simulink model "Vehicle_Model_WIP"  (R2019b)
settings: Solver=FixedStepDiscrete  StartTime=0.0  StopTime=Simulink.t_end  FixedStep=Simulink.dt  RelTol=1e-3
undefined symbols (not defined in the file): BRK, BTRRAD, CHLR, CHRG, DCDC, DiscIntNeverNeededParam, FAN, INV, MTR, PTRAD, PUMP, Settings, TRSM, Vehicle, VHCL, WHL
libraries: simulink x8, EV_cooling x6, EV_VLD x5, EV_ePWT x5
(part 1 of 5)
settings Model: SimulationMode=accelerator  Creator=matteo.yon  LastModifiedBy=matteo.paganini
settings DataIOCC: ReturnWorkspaceOutputs=off
settings DebuggingCC: ArithmeticOperatorsInVariantConditions=warning
settings SFSimCC: SimUseLocalCustomCode=off  CustomCodeUndefinedFunction=UseInterfaceOnly
settings RTWCC: RTWUseLocalCustomCode=off

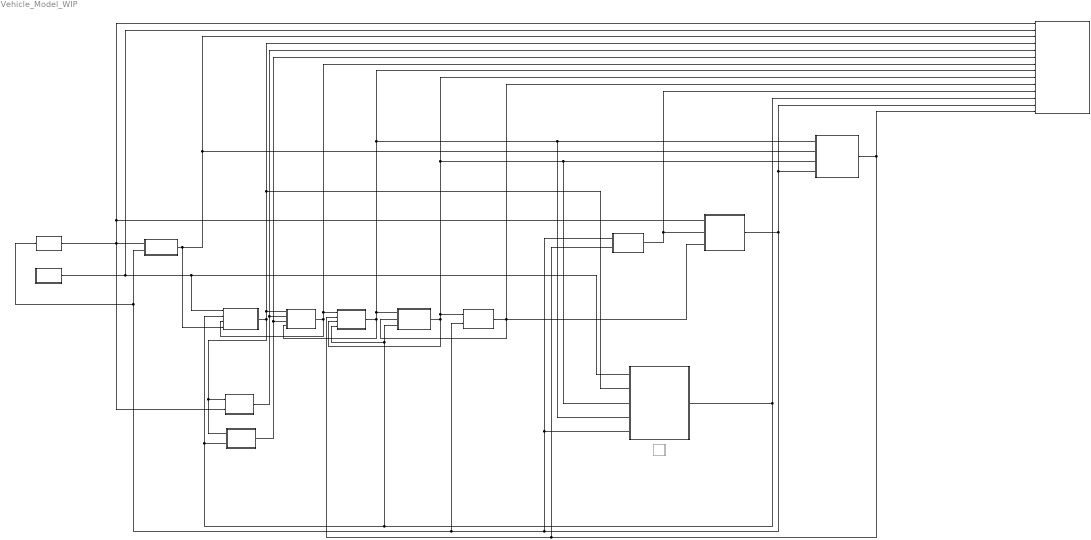
== system Vehicle_Model_WIP ==
  note: Cooling system
  note: Plot Results and Data Logging
  note: Electric Motor
  note: Inverter
  note: Initialization
  note: Battery Pack
  note: Model Input (speed cycle)
  note: Vehicle Longitudinal Dynamics
  note: Driver
  note: Transmission
  note: Electric Power Train Model
  note: Brake system
  note: Vehicle Control Unit
  note: DC Line
  note: DCDC
  note: Electric Vehicle Model
  note: Charger
  BRK : Subsystem
  BTR : Subsystem
  CHRG : Subsystem
  CS : Subsystem
  DC : Subsystem
  DCDC : Subsystem
  DRV : Subsystem
  INIT : Subsystem
  INPT : Subsystem
  INV : Subsystem
  MTR : Subsystem
  Plot Results and Data Logging : Subsystem
  TRSM : Subsystem
  VCU : Subsystem
  VLD : Subsystem
  old cooling : Subsystem  Commented=on
  wires:
  INPT/1(INPT) -> Plot Results and Data Logging/1(INPT), VLD/1(INPT), CHRG/2(INPT), DRV/1(INPT)  "INPT"
  BTR/1(BTR) -> DCDC/1(BTR), CHRG/1(BTR), DC/1(BTR), Plot Results and Data Logging/4(BTR), CS/2(BTR)
  DRV/1(DRV) -> BTR/4(DRV), Plot Results and Data Logging/3(DRV), VCU/2(DRV)  "DRV"
  INV/1(INV) -> MTR/1(INV), Plot Results and Data Logging/8(INV), CS/4(INV), VCU/1(INV), DC/4(INV)
  MTR/1(MTR) -> Plot Results and Data Logging/9(MTR), CS/3(MTR), VCU/3(MTR), TRSM/1(MRT), INV/3(MTR)
  TRSM/1(TRSM) -> Plot Results and Data Logging/10(TRSM), VLD/3(TRSM), MTR/2(TRSM)  "TRSM"
  BRK/1(BRK) -> Plot Results and Data Logging/11(BRK), VLD/2(BRK)
  INIT/1(INIT) -> CS/1(INIT), BTR/1(INIT), Plot Results and Data Logging/2(INIT)  "INIT"
  DC/1(DC) -> BTR/3(DC), Plot Results and Data Logging/7(DC), INV/1(DC)
  VLD/1(VLD) -> Plot Results and Data Logging/13(VLD), VCU/4(VLD), TRSM/2(VLD), DRV/2(VLD), INPT/1(VLD), BRK/1(VLD), CS/5(VLD)  "LVD"
  VCU/1(VCU) -> BRK/2(VCU), INV/2(VCU), Plot Results and Data Logging/14(VCU)  "VCU"
  DCDC/1(DCDC) -> Plot Results and Data Logging/6(DCDC), DC/3(DCDC)
  CHRG/1(CHRG) -> DC/2(CHRG), Plot Results and Data Logging/5(CHRG)
  CS/1(CS) -> Plot Results and Data Logging/12(CS), INV/4(CS), MTR/3(CS), BTR/2(CS), DCDC/2(CS)

== system Vehicle_Model_WIP/BRK ==
  note: Rear Brake
  note: Front Brake
  note: Inverter model:
      | Input: Brake cmd from VCU model.
      | Output: Brake torque.
  VLD : Inport
  VCU : Inport  Port=2
  Add3 : Sum
  Bus Creator : BusCreator  Inputs=6
  Bus Selector2 : BusSelector  OutputSignals=VLD_nWhlFr_rpm,VLD_nWhlRr_rpm,VLD_vActVhcl_kph
  Bus Selector3 : BusSelector  OutputSignals=VCU_rBrkCmdFrt,VCU_rBrkCmdRr
  Constant1 : Constant  Value=Simulink.INIT_TSys_degC
  Constant2 : Constant  Value=Simulink.INIT_TSys_degC
  Discrete-Time Integrator : DiscreteIntegrator  IntegratorMethod=Integration: Trapezoidal  gainval=1e-3/3600  SampleTime=-1  ICPrevOutput=DiscIntNeverNeededParam  ICPrevScaledInput=DiscIntNeverNeededParam
  Front BRAKE : EV_VLD/BRAKE  MxTrq_Nm=BRK.Front.Mx_Torque_Nm/2  eff=BRK.Front.Eff_BrkSys  HC_disc=BRK.Front.Cdisc_JpK  T_env_degC=Simulink.INIT_TEnv_degC  R_StoC_KpW=0.0035*0.8  HTC_v_bp=BRK.Front.HTC_v_bp  HTC_map=BRK.Front.HTC_map
      settings: SourceProductName=EV_lib
  Gain{1..4} (4 alike) : Gain  Gain=2
  Rear BRAKE : EV_VLD/BRAKE  MxTrq_Nm=BRK.Rear.Mx_Torque_Nm/2  eff=BRK.Rear.Eff_BrkSys  HC_disc=BRK.Rear.Cdisc_JpK  T_env_degC=Simulink.INIT_TEnv_degC  R_StoC_KpW=0.0035*0.8  HTC_v_bp=BRK.Rear.HTC_v_bp  HTC_map=BRK.Rear.HTC_map
      settings: SourceProductName=EV_lib
  Scope1 : Scope  NumInputPorts=2
  BRK : Outport  VectorParamsAs1DForOutWhenUnconnected=off
  wires:
  Bus Creator/1 -> BRK/1
  VCU/1 -> Bus Selector3/1
  VLD/1 -> Bus Selector2/1
  [BRK_TActFrt_Nm] -> Bus Creator/1  "BRK_TActFrt_Nm"
  [BRK_TActRr_Nm] -> Bus Creator/2  "BRK_TActRr_Nm"
  Bus Selector2/1 -> [VLD_nWhlFr_rpm]  "<VLD_nWhlFr_rpm>"
  Bus Selector2/2 -> [VLD_nWhlRr_rpm]  "<VLD_nWhlRr_rpm>"
  Bus Selector3/2 -> [VCU_rBrkCmdRr]  "<VCU_rBrkCmdRr>"
  Bus Selector3/1 -> [VCU_rBrkCmdFrt]  "<VCU_rBrkCmdFrt>"
  [BRK_PwrFrt_W] -> Add3/1
  [BRK_PwrRr_W] -> Add3/2
  Add3/1 -> Discrete-Time Integrator/1, [BRK_Pwr_W]
  [BRK_Pwr_W] -> Bus Creator/3  "BRK_Pwr_W"
  Discrete-Time Integrator/1 -> [BRK_E_kWh]
  [BRK_E_kWh] -> Bus Creator/4  "BRK_E_kWh"
  Front BRAKE/2 -> Gain2/1
  Front BRAKE/1 -> Gain3/1
  [VLD_nWhlFr_rpm] -> Front BRAKE/2
  Bus Selector2/3 -> [VLD_vActVhcl_kph]  "<VLD_vActVhcl_kph>"
  [VLD_vActVhcl_kph] -> Front BRAKE/3
  Constant1/1 -> Front BRAKE/4
  Front BRAKE/3 -> Scope1/1, [BRK_TFrt_degC]
  Rear BRAKE/1 -> Gain1/1
  Rear BRAKE/3 -> [BRK_TRr_degC], Scope1/2
  Rear BRAKE/2 -> Gain4/1
  Constant2/1 -> Rear BRAKE/4
  [VLD_nWhlRr_rpm] -> Rear BRAKE/2
  [VLD_vActVhcl_kph] -> Rear BRAKE/3
  [BRK_TFrt_degC] -> Bus Creator/5  "BRK_TFrt_degC"
  [BRK_TRr_degC] -> Bus Creator/6  "BRK_TRr_degC"
  Gain2/1 -> [BRK_PwrFrt_W]
  Gain3/1 -> [BRK_TActFrt_Nm]
  [VCU_rBrkCmdFrt] -> Front BRAKE/1
  Gain1/1 -> [BRK_TActRr_Nm]
  Gain4/1 -> [BRK_PwrRr_W]
  [VCU_rBrkCmdRr] -> Rear BRAKE/1

== system Vehicle_Model_WIP/BTR ==
  INIT : Inport
  CS : Inport  Port=2
  DC : Inport  Port=3
  DRV : Inport  Port=4
  1-D Lookup Table1 : Lookup_n-D  NumberOfTableDimensions=1  BreakpointsForDimension1=[0 20 50 100]  Table=[0 0 1 1]  InternalRulePriority=Speed  RndMeth=Simplest  InputSameDT=on
  1-D Lookup Table2 : Lookup_n-D  NumberOfTableDimensions=1  BreakpointsForDimension1=[0 60 80 100]  Table=[250 250 0 0]*1e3  InternalRulePriority=Speed  RndMeth=Simplest  InputSameDT=on
  Battery : EV_ePWT/Battery  n_series=BTR.cell_p.n_series  n_parallel=BTR.cell_p.n_parallel  weight_ratio=0.7  C_cell_Ah=BTR.cell_p.capacity_nom  V_nominal=BTR.cell_p.voltage_nom  R_contact=0  V_low=BTR.cell_p.Vmin  V_up=BTR.cell_p.Vmax  R_th_KpW=BTR.cell_p.R_th  c_th=BTR.cell_p.c_th  weight=BTR.cell_p.weight  VoC_map=BTR.cell_p.VOC  VoC_SoC_bp=BTR.cell_p.SOC_bp_VOC  VoC_Temp_bp=BTR.cell_p.Temp_bp_VOC  VoC_C_bp=BTR.cell_p.C_bp  R0_map=BTR.cell_p.R0  R0_SoC_bp=BTR.cell_p.SOC_bp  R0_Temp_bp=BTR.cell_p.Temp_bp  R0_i_bp=BTR.cell_p.I_bp  R0_C_bp=BTR.cell_p.C_bp  R1_map=BTR.cell_p.R1  R1_SoC_bp=BTR.cell_p.SOC_bp  R1_Temp_bp=BTR.cell_p.Temp_bp  R1_i_bp=BTR.cell_p.I_bp  R1_C_bp=BTR.cell_p.C_bp  tau1_map=BTR.cell_p.tau  tau1_SoC_bp=BTR.cell_p.SOC_bp  tau1_Temp_bp=BTR.cell_p.Temp_bp  tau1_i_bp=BTR.cell_p.I_bp  tau1_C_bp=BTR.cell_p.C_bp  Limit_temp_bp=[-30 -10 0 55 57 58]  Limit_map=[0 0.2 1 1 0.2 0]  max_peak_crate=10  max_crate=5  peak_time=30
  Bus Creator : BusCreator  Inputs=13
  Bus Selector : BusSelector  OutputSignals=INIT_TSys_degC,INIT_SocBtr_Pct
  Bus Selector1 : BusSelector  OutputSignals=DC_PBtrReq_W
  Bus Selector2 : BusSelector  OutputSignals=CS_BTR_TWtrOut_degC,CS_BTR_dm_kgps
  Bus Selector3 : BusSelector  OutputSignals=DRV_FC_enable
  Delay1 : Delay  DelayLength=1
  Delay2 : Delay  DelayLength=1  InitialCondition=20000
  Divide : Product  Inputs=*/
  FuelCells : Subsystem
  Gain : Gain  Gain=100
  Gain1 : Gain  Gain=1/100
  Gain2 : Gain  Gain=1e-3
  Mux : Mux  Inputs=2
  Product : Product
  Scope : Scope  NumInputPorts=2
  Sum : Sum  Inputs=-+|
  Sum1 : Sum  Inputs=++|
  Tentativo picchi richiesta FC : Lookup_n-D  NumberOfTableDimensions=1  BreakpointsForDimension1=[0 40 45 100]  Table=[250 250 0 0]*1e3  InternalRulePriority=Speed  RndMeth=Simplest  InputSameDT=on
  Terminator : Terminator
  Terminator2 : Terminator
  To Workspace : ToWorkspace  VariableName=actPower_W  SaveFormat=Timeseries  SampleTime=-1
  reset_time : Constant  Value=1e6
  BTR : Outport  VectorParamsAs1DForOutWhenUnconnected=off
  wires:
  [INIT_SocBtr_Pct] -> Gain1/1
  [BTR_VPackEst_V] -> Bus Creator/2  "BTR_VPackEst_V"
  [BTR_iPackEst_A] -> Bus Creator/1  "BTR_iPackEst_A"
  [BTR_PPackEst_W] -> Bus Creator/3  "BTR_PPackEst_W"
  [BTR_SocPack_Ptc] -> Bus Creator/4  "BTR_SocPack_Ptc"
  [BTR_PMxDsch_W] -> Bus Creator/5  "BTR_PMxDsch_W"
  [BTR_PMxChrg_W] -> Bus Creator/6  "BTR_PMxChrg_W"
  [BTR_TMxCell_degC] -> Bus Creator/7  "BTR_TMxCell_degC"
  [BTR_TMxBsbr_C] -> Bus Creator/8  "BTR_TMxBsbr_C"
  [BTR_TWtrOut_degC] -> Bus Creator/9  "BTR_TWtrOut_degC"
  Bus Creator/1 -> BTR/1
  INIT/1 -> Bus Selector/1
  Bus Selector/2 -> [INIT_SocBtr_Pct]  "<INIT_SocBtr_Pct>"
  Bus Selector/1 -> [INIT_TSys_degC]  "<INIT_TSys_degC>"
  DC/1 -> Bus Selector1/1
  Bus Selector1/1 -> [DC_PBtrReq_W]  "<DC_PBtrReq_W>"
  CS/1 -> Bus Selector2/1
  Bus Selector2/1 -> [BCS_TWtrOut_degC]  "<CS_BTR_TWtrOut_degC>"
  Bus Selector2/2 -> [BCS_dm_kgps]  "<CS_BTR_dm_kgps>"
  Delay1/1 -> [BTR_PBtrReq_W], Battery/1
  Battery/3 -> [BTR_PPackEst_W]
  Battery/4 -> [BTR_iPackEst_A]
  Battery/6 -> Gain/1
  Battery/10 -> [BTR_PMxChrg_W]
  Battery/7 -> [BTR_TMxBsbr_C], [BTR_TMxCell_degC]
  Battery/5 -> [BTR_VPackEst_V]
  Gain/1 -> Scope/2, [BTR_SocPack_Ptc]  "HVB_SOC"
  [INIT_TSys_degC] -> Battery/3
  Battery/1 -> Terminator2/1
  Gain1/1 -> Battery/2
  Battery/2 -> [BTR_EPack_kWh]
  [BTR_EPack_kWh] -> Bus Creator/10  "BTR_EPack_kWh"
  reset_time/1 -> Battery/6
  Battery/11 -> [BTR_HR_pack_W]
  [BTR_HR_pack_W] -> Bus Creator/11  "BTR_HR_pack_W"
  [BCS_dm_kgps] -> Battery/4
  [BCS_TWtrOut_degC] -> Battery/5
  Battery/8 -> [BTR_TWtrOut_degC]
  [DC_PBtrReq_W] -> Sum/2
  Sum/1 -> Mux/2, Delay1/1  "HVB_P"
  FuelCells/1(actPower_W) -> To Workspace/1, Mux/1, [BTR_FCPower_W], Sum/1  "FC_P"
  [BTR_FCPower_W] -> Bus Creator/12  "BTR_FCPower_W"
  Battery/9 -> Product/2
  Sum1/1 -> [BTR_PMxDsch_W]
  [BTR_FCPower_W] -> Delay2/1
  Delay2/1 -> Sum1/1
  1-D Lookup Table2/1 -> FuelCells/1(reqPower_W)
  [BTR_SocPack_Ptc] -> 1-D Lookup Table2/1
  [BTR_PBtrReq_W] -> Bus Creator/13  "BTR_PBtrReq_W"
  Mux/1 -> Scope/1
  [BTR_SocPack_Ptc] -> 1-D Lookup Table1/1
  Product/1 -> Sum1/2
  1-D Lookup Table1/1 -> Product/1
  [BTR_EPack_kWh] -> Divide/2
  Divide/1 -> Terminator/1  "BTR_PDsch_C"
  [BTR_PPackEst_W] -> Gain2/1
  Gain2/1 -> Divide/1
  DRV/1 -> Bus Selector3/1
  Bus Selector3/1 -> [DRV_FC_enable]  "<DRV_FC_enable>"
  [DRV_FC_enable] -> FuelCells/2(DRV_FC_enable)

== system Vehicle_Model_WIP/CHRG ==
  note: Charger model (only efficiency).
      | Input: charge power.
      | Output: charge power to the DC line.
  BTR : Inport
  INPT : Inport  Port=2
  1-D Lookup Table : Lookup_n-D  NumberOfTableDimensions=1  BreakpointsForDimension1=[-20 0 5 90]  Table=-[250 350 450 450]  InternalRulePriority=Speed  RndMeth=Simplest  InputSameDT=on
  1/C : Gain  Gain=1/1516.15
  1/R_toair : Gain  Gain=1/0.5
  Abs : Abs
  Bus Creator : BusCreator  Inputs=3
  Bus Selector1 : BusSelector  OutputSignals=INPT_PwrChrg_W
  Bus Selector2 : BusSelector  OutputSignals=BTR_VPackEst_V,BTR_PMxChrg_W
  Constant3 : Constant  Value=CHRG.Efficiency
  Discrete-Time Integrator : DiscreteIntegrator  InitialConditionSource=external  InitialCondition=23  SampleTime=-1  ICPrevOutput=DiscIntNeverNeededParam  ICPrevScaledInput=DiscIntNeverNeededParam
  Divide1 : Product  Inputs=*/
  Divide2 : Product  Inputs=**
  Divide3 : Product  Inputs=*/
  Divide4 : Product  Inputs=*/
  MinMax1 : MinMax  Function=max  Inputs=3
  MinMax2 : MinMax  Function=max  Inputs=2
  R_joule : Gain  Gain=0.001
  Scope : Scope
  Scope1 : Scope
  Scope2 : Scope
  Square : Math  Operator=square  SignedPower=off  SaturateOnIntegerOverflow=on
  Subtract : Sum  Inputs=+-
  Subtract1 : Sum  Inputs=+-
  Subtract2 : Sum  Inputs=-+
  Switch : Switch  Criteria=u2 > Threshold  Threshold=1e4
  T_ambient : Constant  Value=Simulink.INIT_TEnv_degC
  T_ref : Constant  Value=90
  CHRG : Outport  VectorParamsAs1DForOutWhenUnconnected=off
  wires:
  [CHRG_Pwr_W] -> Bus Creator/1  "CHRG_Pwr_W"
  Bus Selector1/1 -> [INPT_PwrChrg_W]  "<INPT_PwrChrg_W>"
  Bus Creator/1 -> CHRG/1
  INPT/1 -> Bus Selector1/1
  Constant3/1 -> [CHRG_rEff]
  [T_port_degC] -> Bus Creator/3  "CHRG_Tport_degC"
  BTR/1 -> Bus Selector2/1
  Bus Selector2/1 -> [BTR_VPackEst_V]  "<BTR_VPackEst_V>"
  Square/1 -> R_joule/1
  [T_port_degC] -> Subtract1/1
  1/R_toair/1 -> Subtract/2
  T_ambient/1 -> Discrete-Time Integrator/2, Subtract1/2
  Subtract1/1 -> 1/R_toair/1  "q_dot"
  R_joule/1 -> Subtract/1
  Subtract/1 -> 1/C/1  "q_dot"
  1/C/1 -> Discrete-Time Integrator/1  "dT"
  Discrete-Time Integrator/1 -> Scope2/1, [T_port_degC]  "T"
  Bus Selector2/2 -> [BTR_PMxChrg_W]  "<BTR_PMxChrg_W>"
  [CHRG_iAct_A] -> Square/1  "iChrg_A"
  [CHRG_iAct_A] -> Bus Creator/2  "CHRG_iAct_A"
  [T_port_degC] -> Subtract2/1
  T_ref/1 -> Subtract2/2
  Subtract2/1 -> 1-D Lookup Table/1
  [BTR_VPackEst_V] -> Divide1/2
  [BTR_PMxChrg_W] -> Divide1/1
  Divide1/1 -> MinMax1/1  "iMxChrg_A"
  1-D Lookup Table/1 -> MinMax1/2
  MinMax1/1 -> [CHRG_iAct_A], Scope1/1
  Divide2/1 -> [CHRG_Pwr1_W]
  [CHRG_iAct_A] -> Divide2/1
  [BTR_VPackEst_V] -> Divide2/2
  [INPT_PwrChrg_W] -> Divide3/1
  [BTR_VPackEst_V] -> Divide3/2
  Divide3/1 -> MinMax1/3  "INPT_iChrg_A"
  [CHRG_Pwr1_W] -> Switch/1, Abs/1
  Abs/1 -> Switch/2
  Switch/1 -> Scope/1, [CHRG_Pwr_W]
  [INPT_PwrChrg_W] -> Divide4/1
  [CHRG_rEff] -> Divide4/2
  Divide4/1 -> MinMax2/1
  MinMax2/1 -> Switch/3
  [BTR_PMxChrg_W] -> MinMax2/2

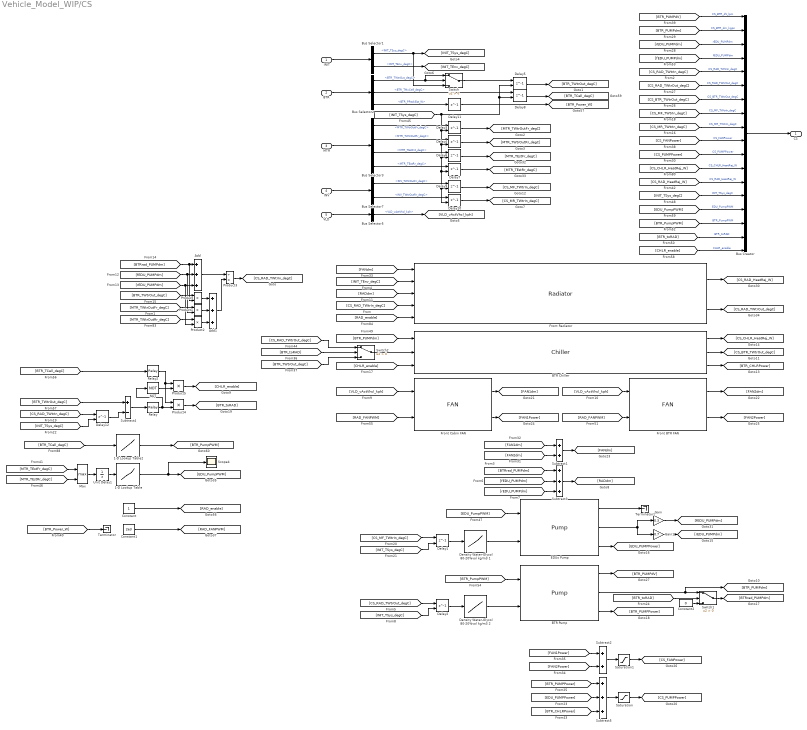
== system Vehicle_Model_WIP/CS ==
  INIT : Inport
  BTR : Inport  Port=2
  MTR : Inport  Port=3
  INV : Inport  Port=4
  VLD : Inport  Port=5
  1-D Lookup Table : Lookup_n-D  NumberOfTableDimensions=1  BreakpointsForDimension1=[0 60 100 120 150]  Table=[1000 1000 3500 5500 5500]  InternalRulePriority=Speed  RndMeth=Simplest  InputSameDT=on
  1-D Lookup Table2 : Lookup_n-D  NumberOfTableDimensions=1  BreakpointsForDimension1=[0 35 50 55 70]  Table=[2000 2000 4000 5500 5500]  InternalRulePriority=Speed  RndMeth=Simplest  InputSameDT=on
  Add : Sum  Inputs=+++
  Add1 : Sum  Inputs=+++
  BTR Chiller : EV_cooling/Chiller  dm_water_bp=(0:0.05:0.25)'  T_water_bp=0:10:40  HR_map=[0,0,0,0,0;0,300,600,900,0;0,600,1200,1800,0;0,900,1800,2700,0;0,1200,2400,3600,0;0,1500,3000,4500,0]  COP=2.5
      settings: SourceProductName=EV_lib
  BTR Pump : EV_cooling/Pump  RPM_bp=PUMP.Front.BCS_RPM_bp1  dV_map=PUMP.Front.BCS_dV  power_map=PUMP.Front.BCS_power
      settings: SourceProductName=EV_lib
  Bus Creator : BusCreator  Inputs=18
  Bus Selector1 : BusSelector  OutputSignals=INIT_TSys_degC,INIT_TEnv_degC
  Bus Selector2 : BusSelector  OutputSignals=BTR_TWtrOut_degC,BTR_TMxCell_degC,BTR_PPackEst_W
  Bus Selector3 : BusSelector  OutputSignals=MTR_TWtrOutFr_degC,MTR_TWtrOutRr_degC,MTR_TEstFrt_degC,MTR_TEstRr_degC
  Bus Selector5 : BusSelector  OutputSignals=VLD_vActVhcl_kph
  Bus Selector7 : BusSelector  OutputSignals=INV_TWtrOutFr_degC,INV_TWtrOutRr_degC
  Constant : Constant
  Constant1 : Constant  Value=2e3
  Constant2 : Constant  Value=0
  Delay{1..10,12} (11 alike) : Delay  DelayLength=1  InitialConditionSource=Input port
      settings: InputPortMap=u0,p4
  Delay11 : Delay  DelayLength=1
  Density Water-Glycol 80-20%vol kg/m3 1 : Lookup_n-D  NumberOfTableDimensions=1  BreakpointsForDimension1=[-45.56 -17.78 10 37.77 65.55 93.33 121.11 148.88 176.66]  Table=[1.02e+03 1.03e+03 1.03e+03 1.02e+03 9.99e+02 9.85e+02 9.63e+02 9.38e+02 9.11e+02]  ExtrapMethod=Clip  RndMeth=Simplest  InputSameDT=on
  Density Water-Glycol 80-20%vol kg/m3 2 : Lookup_n-D  NumberOfTableDimensions=1  BreakpointsForDimension1=[-45.56 -17.78 10 37.77 65.55 93.33 121.11 148.88 176.66]  Table=[1.02e+03 1.03e+03 1.03e+03 1.02e+03 9.99e+02 9.85e+02 9.63e+02 9.38e+02 9.11e+02]  ExtrapMethod=Clip  RndMeth=Simplest  InputSameDT=on
  EDUs Pump : EV_cooling/Pump  RPM_bp=PUMP.Front.PWT_RPM_bp1  dV_map=PUMP.Front.PWT_dV  power_map=PUMP.Front.PWT_power
      settings: SourceProductName=EV_lib
  Front BTR FAN : EV_cooling/FAN  speed_bp=FAN.Front.f15_V_bp  RPM_bp=FAN.Front.f15_RPM_bp  dm_map=FAN.Front.f15_dm_air  power_map=FAN.Front.f15_power
      settings: SourceProductName=EV_lib
  Front Cabin FAN : EV_cooling/FAN  speed_bp=FAN.Front.f11_V_bp  RPM_bp=FAN.Front.f11_RPM_bp  dm_map=FAN.Front.f11_dm_air  power_map=FAN.Front.f11_power
      settings: SourceProductName=EV_lib
  Front Radiator : EV_cooling/Radiator  dm_water_bp=RAD.Front.FC_dmw_bp  dm_air_bp=RAD.Front.FC_dma_bp  normHR_map=RAD.Front.FC_normHR  FrontSurf=RAD.Front.ABTR_m2
      settings: SourceProductName=EV_lib
  Gain : Gain  Gain=0.3
  Gain1 : Gain  Gain=0.7
  Max : MinMax  Function=max  Inputs=2
  NOT : Logic  Operator=NOT  IconShape=distinctive  AllPortsSameDT=off  OutDataTypeStr=boolean
  Product{,1..2,4..5} (5 alike) : Product
  Product3 : Product  Inputs=/*
  Relay : Relay  OnSwitchValue=2  OffSwitchValue=-2
  Relay2 : Relay  OnSwitchValue=31  OffSwitchValue=29
  Saturation : Saturate  UpperLimit=0  LowerLimit=0
  Saturation1 : Saturate  UpperLimit=0  LowerLimit=0
  Scope4 : Scope
  Subtract1 : Sum
  Subtract2 : Sum
  Subtract3 : Sum  Inputs=+++
  Subtract4 : Sum  Inputs=+-
  Subtract5 : Sum  Inputs=+++
  Switch : Switch  Criteria=u2 > Threshold
  Switch1 : Switch  Criteria=u2 > Threshold
  Switch2 : Switch  Criteria=u2 > Threshold
  Terminator : Terminator
  Terminator2 : Terminator
  Unit Delay1 : UnitDelay  InitialCondition=Settings.INIT_TSys_degC  SampleTime=-1  HasFrameUpgradeWarning=on
  CS : Outport
  wires:
  Bus Selector1/2 -> [INIT_TEnv_degC]  "<INIT_TEnv_degC>"
  INIT/1 -> Bus Selector1/1
  Bus Selector1/1 -> Switch/3, [INIT_TSys_degC]  "<INIT_TSys_degC>"
  BTR/1 -> Bus Selector2/1
  MTR/1 -> Bus Selector3/1
  Bus Selector5/1 -> [VLD_vActVhcl_kph]  "<VLD_vActVhcl_kph>"
  VLD/1 -> Bus Selector5/1
  [CS_RAD_TWtrIn_degC] -> Front Radiator/4
  Bus Creator/1 -> CS/1
  [CS_MR_TWtrIn_degC] -> Bus Creator/9  "CS_MR_TWtrIn_degC"
  [CS_MF_TWtrIn_degC] -> Bus Creator/8  "CS_MF_TWtrIn_degC"
  [INIT_TSys_degC] -> Delay1/2
  [CS_MF_TWtrIn_degC] -> Delay1/1
  Delay1/1 -> Density Water-Glycol 80-20%vol kg/m3 1/1
  [EDU_PumpPWM] -> EDUs Pump/1
  EDUs Pump/2 -> Gain/1, Gain1/1
  EDUs Pump/3 -> [EDU_PUMPPower]
  BTR Pump/3 -> [BTR_PUMPPower]
  Delay2/1 -> Density Water-Glycol 80-20%vol kg/m3 2/1
  [INIT_TSys_degC] -> Delay2/2
  [CS_RAD_TWtrOut_degC] -> Delay2/1
  [CS_RAD_TWtrOut_degC] -> Bus Creator/6  "CS_RAD_TWtrOut_degC"
  [rEDU_PUMPdm] -> Bus Creator/3  "rEDU_PUMPdm"
  [BTR_PUMPdm] -> Bus Creator/2  "CS_BTR_dm_kgps"
  [BTR_PUMPPower] -> Subtract5/1
  [EDU_PUMPPower] -> Subtract5/2
  Subtract5/1 -> Saturation/1
  [CS_PUMPPower] -> Bus Creator/11  "CS_PUMPPower"
  Front BTR FAN/1 -> [FAN2dm]
  [FAN1dm] -> Subtract1/1
  [FAN2dm] -> Subtract1/2
  Subtract1/1 -> [FANdm]
  [FANdm] -> Front Radiator/1
  Front Radiator/1 -> [CS_RAD_HeatRej_W]
  Front BTR FAN/2 -> [FAN2Power]
  [FAN1Power] -> Subtract2/1
  [FAN2Power] -> Subtract2/2
  Subtract2/1 -> Saturation1/1
  [CS_FANPower] -> Bus Creator/10  "CS_FANPower"
  [BTR_PUMPdV] -> Bus Creator/1  "CS_BTR_dV_lpm"
  Bus Selector3/1 -> Delay3/1  "<MTR_TWtrOutFr_degC>"
  Bus Selector3/2 -> Delay4/1  "<MTR_TWtrOutRr_degC>"
  Delay3/1 -> [MTR_TWtrOutFr_degC]
  Delay4/1 -> [MTR_TWtrOutRr_degC]
  [CS_RAD_HeatRej_W] -> Bus Creator/13  "CS_RAD_HeatRej_W"
  Front Cabin FAN/2 -> [FAN1Power]
  Front Cabin FAN/1 -> [FAN1dm]
  EDUs Pump/1 -> Terminator2/1
  BTR Pump/1 -> [BTR_PUMPdV]
  Switch/1 -> Delay5/1
  [INIT_TSys_degC] -> Delay8/2, Delay5/2, Delay10/2, Delay9/2, Delay7/2, Delay6/2, Delay4/2, Delay3/2
  Delay5/1 -> [BTR_TWtrOut_degC]
  Delay7/1 -> [MTR_TEstRr_degC]
  Delay6/1 -> [MTR_TEstFr_degC]
  Bus Selector3/4 -> Delay7/1  "<MTR_TEstRr_degC>"
  Bus Selector3/3 -> Delay6/1  "<MTR_TEstFrt_degC>"
  [INIT_TEnv_degC] -> Front Radiator/2
  [RADdm] -> Front Radiator/3
  Density Water-Glycol 80-20%vol kg/m3 1/1 -> EDUs Pump/2
  Density Water-Glycol 80-20%vol kg/m3 2/1 -> BTR Pump/2
  [VLD_vActVhcl_kph] -> Front Cabin FAN/1
  [VLD_vActVhcl_kph] -> Front BTR FAN/1
  [BTR_PumpPWM] -> BTR Pump/1
  [RAD_FANPWM] -> Front Cabin FAN/2
  [RAD_FANPWM] -> Front BTR FAN/2
  Gain/1 -> [fEDU_PUMPdm]
  Gain1/1 -> [rEDU_PUMPdm]
  [fEDU_PUMPdm] -> Bus Creator/4  "fEDU_PUMPdm"
  INV/1 -> Bus Selector7/1
  Delay10/1 -> [CS_MR_TWtrIn_degC]
  Bus Selector7/1 -> Delay9/1  "<INV_TWtrOutFr_degC>"
  Bus Selector7/2 -> Delay10/1  "<INV_TWtrOutRr_degC>"
  [RAD_enable] -> Front Radiator/5
  Front Radiator/2 -> [CS_RAD_TWtrOut_degC]
  [CS_CHLR_HeatRej_W] -> Bus Creator/12  "CS_CHLR_HeatRej_W"
  Max/1 -> Unit Delay1/1
  Unit Delay1/1 -> 1-D Lookup Table/1
  Bus Selector2/3 -> Delay11/1  "<BTR_PPackEst_W>"
  Bus Selector2/1 -> Switch/1, Switch/2  "<BTR_TWtrOut_degC>"
  Bus Selector2/2 -> Delay8/1  "<BTR_TMxCell_degC>"
  Delay8/1 -> [BTR_TCell_degC]
  Delay11/1 -> [BTR_Power_W]
  [BTR_TCell_degC] -> 1-D Lookup Table2/1
  1-D Lookup Table2/1 -> [BTR_PumpPWM]
  1-D Lookup Table/1 -> [EDU_PumpPWM], Scope4/1
  Constant/1 -> [RAD_enable]
  Constant1/1 -> [RAD_FANPWM]
  [BTR_Power_W] -> Terminator/1
  Saturation/1 -> [CS_PUMPPower]
  Saturation1/1 -> [CS_FANPower]
  [BTRrad_PUMPdm] -> Subtract3/1
  [fEDU_PUMPdm] -> Subtract3/2
  [rEDU_PUMPdm] -> Subtract3/3
  Subtract3/1 -> [RADdm]
  [CS_RAD_TWtrIn_degC] -> Bus Creator/5  "CS_RAD_TWtrIn_degC"
  [BTR_TWtrOut_degC] -> Product/1
  [MTR_TWtrOutFr_degC] -> Product1/1
  [MTR_TWtrOutRr_degC] -> Product2/1
  [rEDU_PUMPdm] -> Product2/2, Add/3
  [fEDU_PUMPdm] -> Product1/2, Add/2
  [BTRrad_PUMPdm] -> Product/2, Add/1
  Product/1 -> Add1/1
  Product2/1 -> Add1/3
  Product1/1 -> Add1/2
  Add/1 -> Product3/1
  Add1/1 -> Product3/2
  Product3/1 -> [CS_RAD_TWtrIn_degC]
  [MTR_TEstFr_degC] -> Max/1
  [MTR_TEstRr_degC] -> Max/2
  Delay9/1 -> [CS_MF_TWtrIn_degC]
  [CS_RAD_TWtrIn_degC] -> Delay12/1
  [INIT_TSys_degC] -> Delay12/2
  Delay12/1 -> Subtract4/2
  Subtract4/1 -> Relay/1
  [BTR_toRAD] -> Switch1/2
  BTR Pump/2 -> [BTR_PUMPdm], Switch1/1
  Constant2/1 -> Switch1/3
  Switch1/1 -> [BTRrad_PUMPdm]
  [CS_BTR_TWtrOut_degC] -> Bus Creator/7  "CS_BTR_TWtrOut_degC"
  [BTR_toRAD] -> Switch2/2
  [BTR_TWtrOut_degC] -> Switch2/3
  [CS_RAD_TWtrOut_degC] -> Switch2/1
  BTR Chiller/2 -> [CS_BTR_TWtrOut_degC]
  BTR Chiller/3 -> [BTR_CHLRPower]
  Switch2/1 -> BTR Chiller/2
  [BTR_CHLRPower] -> Subtract5/3
  [BTR_PUMPdm] -> BTR Chiller/1
  BTR Chiller/1 -> [CS_CHLR_HeatRej_W]
  [BTR_TWtrOut_degC] -> Subtract4/1
  Relay2/1 -> Product4/1, Product5/1
  NOT/1 -> Product5/2
  [BTR_TCell_degC] -> Relay2/1
  Product4/1 -> [BTR_toRAD]
  Relay/1 -> NOT/1, Product4/2
  Product5/1 -> [CHLR_enable]
  [CHLR_enable] -> BTR Chiller/3
  [BTR_toRAD] -> Bus Creator/17  "BTR_toRAD"
  [CHLR_enable] -> Bus Creator/18  "CHLR_enable"
  [INIT_TSys_degC] -> Bus Creator/14  "INIT_TSys_degC"
  [EDU_PumpPWM] -> Bus Creator/15  "EDU_PumpPWM"
  [BTR_PumpPWM] -> Bus Creator/16  "BTR_PumpPWM"

== system Vehicle_Model_WIP/DC ==
  note: DC line model (only efficiency)
      | Take all the power request to battery.
      | To do: Add electrical resistance! (Losses)
  BTR : Inport
  CHRG : Inport  Port=2
  DCDC : Inport  Port=3
  INV : Inport  Port=4
  Add5 : Sum  Inputs=+++
  Bus Creator : BusCreator  Inputs=8
  Bus Selector : BusSelector  OutputSignals=INV_PwrIn_W
  Bus Selector1 : BusSelector  OutputSignals=BTR_PPackEst_W,BTR_PMxDsch_W,BTR_PMxChrg_W,BTR_VPackEst_V
  Bus Selector2 : BusSelector  OutputSignals=DCDC_PwrAux_W
  Bus Selector3 : BusSelector  OutputSignals=CHRG_Pwr_W
  Discrete-Time Integrator : DiscreteIntegrator  IntegratorMethod=Integration: Trapezoidal  gainval=1e-3/3600  SampleTime=-1  ICPrevOutput=DiscIntNeverNeededParam  ICPrevScaledInput=DiscIntNeverNeededParam
  Discrete-Time Integrator1 : DiscreteIntegrator  IntegratorMethod=Integration: Trapezoidal  gainval=1e-3/3600  SampleTime=-1  ICPrevOutput=DiscIntNeverNeededParam  ICPrevScaledInput=DiscIntNeverNeededParam
  Discrete-Time Integrator2 : DiscreteIntegrator  IntegratorMethod=Integration: Trapezoidal  gainval=1e-3/3600  SampleTime=-1  ICPrevOutput=DiscIntNeverNeededParam  ICPrevScaledInput=DiscIntNeverNeededParam
  Saturation : Saturate  UpperLimit=inf  LowerLimit=0
  Saturation1 : Saturate  UpperLimit=0  LowerLimit=-inf
  Scope : Scope  NumInputPorts=3
  DC : Outport  VectorParamsAs1DForOutWhenUnconnected=off
  wires:
  Bus Selector/1 -> [INV_PwrIn_W]  "<INV_PwrIn_W>"
  Bus Creator/1 -> DC/1
  INV/1 -> Bus Selector/1
  Bus Selector1/1 -> [BTR_PPackEst_W]  "<BTR_PPackEst_W>"
  Bus Selector1/4 -> [BTR_VPackEst_V]  "<BTR_VPackEst_V>"
  Bus Selector1/2 -> [BTR_PMxDsch_W]  "<BTR_PMxDsch_W>"
  BTR/1 -> Bus Selector1/1
  Bus Selector1/3 -> [BTR_PMxChrg_W]  "<BTR_PMxChrg_W>"
  [DC_PBtr_W] -> Bus Creator/1  "DC_PBtr_W"
  [DC_PMxDschBtr_W] -> Bus Creator/2  "DC_PMxDschBtr_W"
  [DC_PMxChrg_W] -> Bus Creator/3  "DC_PMxChrg_W"
  [DC_VBtr_V] -> Bus Creator/4  "DC_VBtr_V"
  [INV_PwrIn_W] -> Scope/1, Add5/1
  [DCDC_PwrAux_W] -> Scope/2, Add5/2
  Add5/1 -> [DC_PBtrReq_W]
  [DC_PBtrReq_W] -> Bus Creator/5  "DC_PBtrReq_W"
  [BTR_PPackEst_W] -> [DC_PBtr_W]
  [BTR_PMxDsch_W] -> [DC_PMxDschBtr_W]
  [BTR_PMxChrg_W] -> [DC_PMxChrg_W]
  [BTR_VPackEst_V] -> [DC_VBtr_V]
  DCDC/1 -> Bus Selector2/1
  Bus Selector2/1 -> [DCDC_PwrAux_W]  "<DCDC_PwrAux_W>"
  Bus Selector3/1 -> [CHRG_Pwr_W]  "<CHRG_Pwr_W>"
  CHRG/1 -> Bus Selector3/1
  [CHRG_Pwr_W] -> Scope/3, Add5/3
  Discrete-Time Integrator/1 -> [DC_EBtrPos_kWh]
  [DC_EBtrPos_kWh] -> Bus Creator/7  "DC_EBtrPos_kWh"
  [INV_PwrIn_W] -> Saturation1/1, Saturation/1
  Saturation/1 -> Discrete-Time Integrator/1
  Saturation1/1 -> Discrete-Time Integrator1/1
  Discrete-Time Integrator1/1 -> [DC_EBtrNeg_kWh]
  [DC_EBtrNeg_kWh] -> Bus Creator/8  "DC_EBtrNeg_kWh"
  [DC_PBtr_W] -> Discrete-Time Integrator2/1
  Discrete-Time Integrator2/1 -> Bus Creator/6  "DC_EBtrReq_kWh"

== system Vehicle_Model_WIP/DCDC ==
  note: DCDC model for now an efficiency.
      | Input: power fron 12V, Aux power constant (ex: AC).
      | Output: power for DC line.
  BTR : Inport
  CS : Inport  Port=2
  2-D Lookup Table : Lookup_n-D  BreakpointsForDimension1=DCDC.bp_V  BreakpointsForDimension2=DCDC.bp_power  Table=DCDC.eff'  InternalRulePriority=Speed  RndMeth=Simplest  InputSameDT=on
  Add : Sum  Inputs=4
  Add1 : Sum  Inputs=++++
  Bus Creator : BusCreator  Inputs=5
  Bus Selector : BusSelector  OutputSignals=BTR_VPackEst_V
  Bus Selector3 : BusSelector  OutputSignals=CS_FANPower,CS_PUMPPower
  Constant1 : Constant  Value=VHCL.Aux_PWR_W
  Constant4 : Constant  Value=VHCL.EE12V_PWR_W
  Discrete-Time Integrator : DiscreteIntegrator  gainval=1e-3/3600  SampleTime=-1  ICPrevOutput=DiscIntNeverNeededParam  ICPrevScaledInput=DiscIntNeverNeededParam
  Discrete-Time Integrator1 : DiscreteIntegrator  gainval=1e-3/3600  SampleTime=-1  ICPrevOutput=DiscIntNeverNeededParam  ICPrevScaledInput=DiscIntNeverNeededParam
  Divide{1..2,4..5} (4 alike) : Product  Inputs=*/
  Scope : Scope
  Scope2 : Scope
  Subtract : Sum  Inputs=-+
  Unit Delay : UnitDelay  InitialCondition=430  SampleTime=-1  HasFrameUpgradeWarning=on
  Unit Delay1 : UnitDelay  InitialCondition=750  SampleTime=-1  HasFrameUpgradeWarning=on
  DCDC : Outport  VectorParamsAs1DForOutWhenUnconnected=off
  wires:
  Bus Creator/1 -> DCDC/1
  Constant1/1 -> Add1/3, Divide1/1
  Divide1/1 -> [DCDC_Aux_W]
  [DCDC_rEff] -> Divide1/2
  [DCDC_Aux_W] -> Add/1
  Add/1 -> Discrete-Time Integrator/1, Scope2/1, [DCDC_PwrAux_W]
  [DCDC_PwrAux_W] -> Bus Creator/1  "DCDC_PwrAux_W"
  [DCDC_rEff] -> Bus Creator/2  "DCDC_rEff"
  [CS_FANPower_W] -> Divide2/1
  [DCDC_rEff] -> Divide2/2
  Divide2/1 -> [DCDC_Fan_W]
  [DCDC_Fan_W] -> Add/3
  [DCDC_rEff] -> Divide4/2
  Constant4/1 -> Add1/4, Divide4/1
  Bus Selector3/1 -> [CS_PUMPPower_W]  "<CS_FANPower>"
  CS/1 -> Bus Selector3/1
  Divide5/1 -> [DCDC_Pump_W]
  [DCDC_rEff] -> Divide5/2
  [CS_PUMPPower_W] -> Divide5/1
  [DCDC_Pump_W] -> Add/4
  [DCDC_EE12V_W] -> Add/2
  [DCDC_EE12V_W] -> Bus Creator/3  "DCDC_EE_W"
  [DCDC_EE12V_kWh] -> Bus Creator/4  "DCDC_EE_kWh"
  [DCDC_EAux_kWh] -> Bus Creator/5  "DCDC_EAux_kWh"
  Discrete-Time Integrator1/1 -> [DCDC_EE12V_kWh]
  Divide4/1 -> Discrete-Time Integrator1/1, [DCDC_EE12V_W]
  Discrete-Time Integrator/1 -> Subtract/2
  Subtract/1 -> [DCDC_EAux_kWh]
  [DCDC_EE12V_kWh] -> Subtract/1
  Bus Selector3/2 -> [CS_FANPower_W]  "<CS_PUMPPower>"
  [DCDC_Fan_W] -> Add1/1
  [DCDC_Pump_W] -> Add1/2
  2-D Lookup Table/1 -> Scope/1, [DCDC_rEff]
  Add1/1 -> Unit Delay1/1
  BTR/1 -> Bus Selector/1
  Bus Selector/1 -> [BTR_VPack_V]  "<BTR_VPackEst_V>"
  [BTR_VPack_V] -> Unit Delay/1
  Unit Delay/1 -> 2-D Lookup Table/1
  Unit Delay1/1 -> 2-D Lookup Table/2

== system Vehicle_Model_WIP/DRV ==
  note: Driver model (PID) that follows the required speed with an acceleration and a braking signal.
  INPT : Inport
  VLD : Inport  Port=2
  Bus Creator : BusCreator  Inputs=3
  Bus Selector : BusSelector  OutputSignals=INPT_vReq_kph
  Bus Selector1 : BusSelector  OutputSignals=VLD_vActVhcl_kph
  Driver Model : Subsystem
  Step : Step  Time=20  Before=1  SampleTime=0
  DRV : Outport  VectorParamsAs1DForOutWhenUnconnected=off
  wires:
  INPT/1 -> Bus Selector/1
  Bus Selector/1 -> [INPT_vReq_kph]  "<INPT_vReq_kph>"
  Bus Creator/1 -> DRV/1
  [DRV_rThrottle] -> Bus Creator/1  "DRV_rThrottle"
  [DRV_rBrake] -> Bus Creator/2  "DRV_rBrake"
  Bus Selector1/1 -> [VLD_vActVhcl_kph]  "<VLD_vActVhcl_kph>"
  VLD/1 -> Bus Selector1/1
  [VLD_vActVhcl_kph] -> Driver Model/2(VLD_vActVhcl_kph)
  Driver Model/2(DRV_rBrake) -> [DRV_rBrake]
  Driver Model/1(DRV_rThrottle) -> [DRV_rThrottle]
  Step/1 -> Driver Model/Enable
  [INPT_vReq_kph] -> Driver Model/1(INPT_vReq_kph)
  Driver Model/3(DRV_FC_enable) -> [DRV_FC_enable]
  [DRV_FC_enable] -> Bus Creator/3  "DRV_FC_enable"

== system Vehicle_Model_WIP/INIT ==
  note: Initialization parameters from matlab workspace.
  Bus Creator : BusCreator  Inputs=3
  Constant3 : Constant  Value=Simulink.INIT_TEnv_degC
  Constant7 : Constant  Value=Simulink.INIT_TSys_degC
  Constant8 : Constant  Value=Simulink.INIT_SocBtr_Pct
  INIT : Outport  VectorParamsAs1DForOutWhenUnconnected=off
  wires:
  Constant7/1 -> [INIT_TSys_degC]
  Constant8/1 -> [INIT_SocBtr_Pct]
  Bus Creator/1 -> INIT/1
  [INIT_TSys_degC] -> Bus Creator/1  "INIT_TSys_degC"
  [INIT_SocBtr_Pct] -> Bus Creator/2  "INIT_SocBtr_Pct"
  Constant3/1 -> [INIT_TEnv_degC]
  [INIT_TEnv_degC] -> Bus Creator/3  "INIT_TEnv_degC"

== system Vehicle_Model_WIP/INPT ==
  note: Inputs model from matlab workspace.
  VLD : Inport
  1-D Lookup Table : Lookup_n-D  NumberOfTableDimensions=1  BreakpointsForDimension1=Simulink.Distance(:,2)  Table=Simulink.Speed(:,2)  InternalRulePriority=Speed  RndMeth=Simplest  InputSameDT=on
  Bus Creator : BusCreator  Inputs=3
  Bus Selector : BusSelector  OutputSignals=VLD_lActVhcl_km
  Constant : Constant  Value=0
  Delay : Delay  DelayLength=1
  From Workspace : FromWorkspace  VariableName=Simulink.Speed  SampleTime=0
  From Workspace1 : FromWorkspace  VariableName=Simulink.Slope  SampleTime=0
  From Workspace2 : FromWorkspace  VariableName=Simulink.Chrg_Pwr  SampleTime=0
  Switch : Switch  Criteria=u2 > Threshold
  INPT : Outport  VectorParamsAs1DForOutWhenUnconnected=off
  wires:
  From Workspace1/1 -> [INPT_sReq_Pct]
  Bus Creator/1 -> INPT/1
  [INPT_vReq_kph] -> Bus Creator/1  "INPT_vReq_kph"
  [INPT_sReq_Pct] -> Bus Creator/2  "INPT_sReq_Pct"
  From Workspace/1 -> [INPT_vReq0_kph]
  From Workspace2/1 -> [INPT_PwrChrg_W]
  [INPT_PwrChrg_W] -> Bus Creator/3  "INPT_PwrChrg_W"
  1-D Lookup Table/1 -> Switch/3
  Constant/1 -> Switch/2
  [VLD_lActVhcl_km] -> Delay/1
  [INPT_vReq0_kph] -> Switch/1
  VLD/1 -> Bus Selector/1
  Bus Selector/1 -> [VLD_lActVhcl_km]  "<VLD_lActVhcl_km>"
  Switch/1 -> [INPT_vReq_kph]
  Delay/1 -> 1-D Lookup Table/1

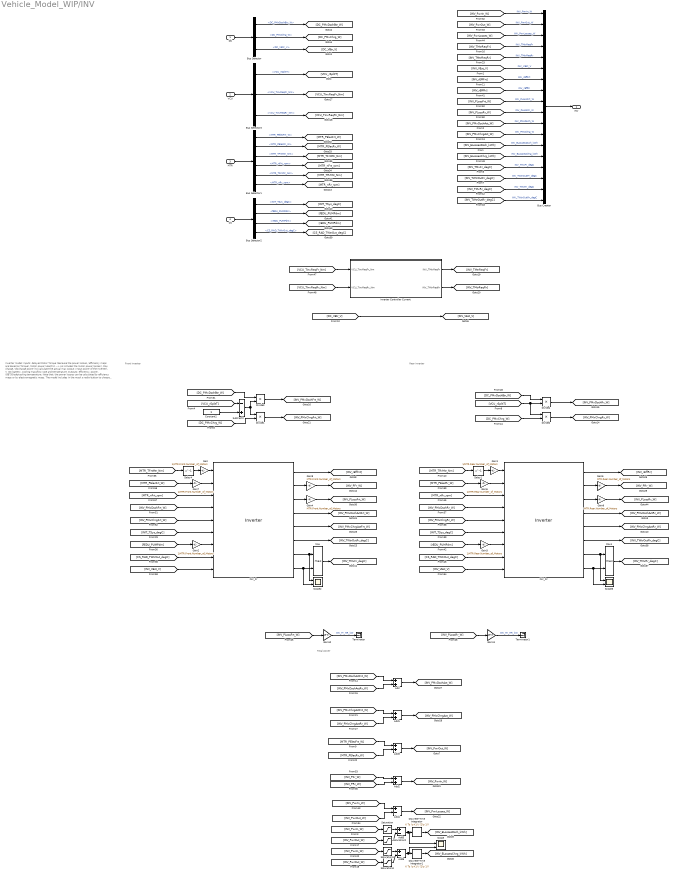
== system Vehicle_Model_WIP/INV ==
  note: Front Inverter
  note: Rear Inverter
  note: Inverter model:
      | Inputs: delayed Motor Torque (because the power losses / efficiency maps are based on Torque), Motor power (electric --> so includes the motor power losses), Max charge / discharge power (to calculate the actual max output / input power of the inverter), V_DC battery, cooling massflow rate and temperature.
      | Outputs: efficiency, power, IGBT/Diode/cooling temperature.
      |
      | Note that: the power losses can be calculated by efficiency maps or by electromagnetic maps. The model includes in the mask a radio-button to choose the method of calculation.
  note: Total power
  DC : Inport
  VCU : Inport  Port=2
  MTR : Inport  Port=3
  CS : Inport  Port=4
  Add{,1..3} (4 alike) : Sum
  Add4 : Sum  Inputs=+-
  Add5 : Sum  Inputs=+-
  Add6 : Sum  Inputs=+-
  Bus Creator : BusCreator  Inputs=18
  Bus Selector : BusSelector  OutputSignals=DC_PMxDschBtr_W,DC_PMxChrg_W,DC_VBtr_V
  Bus Selector1 : BusSelector  OutputSignals=MTR_PElecFrt_W,MTR_PElecRr_W,MTR_TFrtMtr_Nm,MTR_nFrt_rpm,MTR_TRrMtr_Nm,MTR_nRr_rpm
  Bus Selector2 : BusSelector  OutputSignals=INIT_TSys_degC,fEDU_PUMPdm,rEDU_PUMPdm,CS_RAD_TWtrOut_degC
  Bus Selector3 : BusSelector  OutputSignals=VCU_rSplitT,VCU_TInvReqFr_Nm,VCU_TInvReqRr_Nm
  Constant2 : Constant
  Delay1 : Delay  DelayLength=1
  Delay4 : Delay  DelayLength=1
  Discrete-Time Integrator : DiscreteIntegrator  IntegratorMethod=Integration: Trapezoidal  gainval=1e-3/3600  SampleTime=-1  ICPrevOutput=DiscIntNeverNeededParam  ICPrevScaledInput=DiscIntNeverNeededParam
  Discrete-Time Integrator1 : DiscreteIntegrator  IntegratorMethod=Integration: Trapezoidal  gainval=1e-3/3600  SampleTime=-1  ICPrevOutput=DiscIntNeverNeededParam  ICPrevScaledInput=DiscIntNeverNeededParam
  Divide{1..4} (4 alike) : Product
  Gain : Gain  Gain=1/MTR.Front.Number_of_Motors
  Gain1 : Gain  Gain=1/MTR.Rear.Number_of_Motors
  Gain10 : Gain  Gain=1e-3
  Gain11 : Gain  Gain=1e-3
  Gain2 : Gain  Gain=1/MTR.Front.Number_of_Motors
  Gain3 : Gain  Gain=1/MTR.Rear.Number_of_Motors
  Gain4 : Gain  Gain=MTR.Front.Number_of_Motors
  Gain5 : Gain  Gain=1/MTR.Rear.Number_of_Motors
  Gain6 : Gain  Gain=MTR.Rear.Number_of_Motors
  Gain7 : Gain  Gain=1/MTR.Front.Number_of_Motors
  Gain8 : Gain  Gain=MTR.Front.Number_of_Motors
  Gain9 : Gain  Gain=MTR.Rear.Number_of_Motors
  INV_Fr : EV_ePWT/Inverter  C_IGBT=45  R_IGBT=0.038  C_DIO=10  R_DIO=0.070  C_HS=200  R_TIM=0.021  cp_cool=3140  n_poles=6  V_DC_ref=730  RPM_bp=[1000 2000]  torque_bp=[100 200]  Efficiency_map=ones(2,2)*0.98  PL_torque_bp=INV.Front.PLoss_T_bp  PL_RPM_bp=INV.Front.PLoss_n_bp  PL_V_bp=INV.Front.PLoss_V_bp  PL_map=INV.Front.PLoss_table  thermal_mode=from power losses maps
  INV_Rr : EV_ePWT/Inverter  C_IGBT=45  R_IGBT=0.038  C_DIO=10  R_DIO=0.070  C_HS=200  R_TIM=0.021  cp_cool=3140  n_poles=6  V_DC_ref=730  RPM_bp=[1000 2000]  torque_bp=[100 200]  Efficiency_map=ones(2,2)*0.98  PL_torque_bp=INV.Rear.PLoss_T_bp  PL_RPM_bp=INV.Rear.PLoss_n_bp  PL_V_bp=INV.Rear.PLoss_V_bp  PL_map=INV.Rear.PLoss_table  thermal_mode=from power losses maps
  Inverter Controller Current : Subsystem
  Max : MinMax  Function=max  Inputs=2
  Max1 : MinMax  Function=max  Inputs=2
  Saturation : Saturate  UpperLimit=inf  LowerLimit=0
  Saturation1 : Saturate  UpperLimit=0  LowerLimit=-inf
  Saturation2 : Saturate  UpperLimit=inf  LowerLimit=0
  Saturation3 : Saturate  UpperLimit=0  LowerLimit=-inf
  Scope : Scope  NumInputPorts=2
  Scope2 : Scope  NumInputPorts=2
  Scope3 : Scope  NumInputPorts=2
  Subtract2 : Sum  Inputs=-+
  Terminator : Terminator
  Terminator1 : Terminator
  INV : Outport  VectorParamsAs1DForOutWhenUnconnected=off
  wires:
  DC/1 -> Bus Selector/1
  Bus Selector/1 -> [DC_PMxDschBtr_W]  "<DC_PMxDschBtr_W>"
  Bus Selector/2 -> [DC_PMxChrg_W]  "<DC_PMxChrg_W>"
  Bus Creator/1 -> INV/1
  Bus Selector/3 -> [DC_VBtr_V]  "<DC_VBtr_V>"
  [DC_VBtr_V] -> [INV_VEst_V]
  VCU/1 -> Bus Selector3/1
  [DC_PMxDschBtr_W] -> Divide3/1
  [DC_PMxDschBtr_W] -> Divide4/1
  Divide3/1 -> [INV_PMxDschFrt_W]
  Divide4/1 -> [INV_PMxDschRr_W]
  Bus Selector3/2 -> [VCU_TInvReqFr_Nm]  "<VCU_TInvReqFr_Nm>"
  Bus Selector3/3 -> [VCU_TInvReqRr_Nm]  "<VCU_TInvReqRr_Nm>"
  [VCU_TInvReqFr_Nm] -> Inverter Controller Current/1(VCU_TInvReqFr_Nm)
  [VCU_TInvReqRr_Nm] -> Inverter Controller Current/2(VCU_TInvReqRr_Nm)
  Inverter Controller Current/2(INV_TMtrReqRr) -> [INV_TMtrReqRr]
  Inverter Controller Current/1(INV_TMtrReqFr) -> [INV_TMtrReqFr]
  [MTR_PElecRr_W] -> Gain5/1
  [INV_PMxDschRr_W] -> INV_Rr/4
  [INV_PMxChrgRr_W] -> INV_Rr/5
  INV_Rr/5 -> [INV_PMxChrgActRr_W]
  INV_Rr/4 -> [INV_PMxDschActRr_W]
  Add/1 -> [INV_PMxDschAct_W]
  Add1/1 -> [INV_PMxChrgAct_W]
  [INV_PMxChrgActFrt_W] -> Add1/1
  [INV_PMxChrgActRr_W] -> Add1/2
  [INV_PMxDschActRr_W] -> Add/2
  [INV_PMxDschActFrt_W] -> Add/1
  INV_Rr/2 -> Gain6/1
  Add2/1 -> [INV_PwrIn_W]
  MTR/1 -> Bus Selector1/1
  Bus Selector1/1 -> [MTR_PElecFrt_W]  "<MTR_PElecFrt_W>"
  Bus Selector1/2 -> [MTR_PElecRr_W]  "<MTR_PElecRr_W>"
  [MTR_PElecFrt_W] -> Add3/1
  [MTR_PElecRr_W] -> Add3/2
  Add3/1 -> [INV_PwrOut_W]
  [INV_PwrIn_W] -> Bus Creator/1  "INV_PwrIn_W"
  [INV_PwrOut_W] -> Bus Creator/2  "INV_PwrOut_W"
  [INV_PwrIn_W] -> Add4/1
  [INV_PwrOut_W] -> Add4/2
  Add4/1 -> [INV_PwrLosses_W]
  [INV_PwrLosses_W] -> Bus Creator/3  "INV_PwrLosses_W"
  [INV_TMtrReqFr] -> Bus Creator/4  "INV_TMtrReqFr"
  [INV_TMtrReqRr] -> Bus Creator/5  "INV_TMtrReqRr"
  Bus Selector1/3 -> [MTR_TFrtMtr_Nm]  "<MTR_TFrtMtr_Nm>"
  Bus Selector1/4 -> [MTR_nFrt_rpm]  "<MTR_nFrt_rpm>"
  Bus Selector1/6 -> [MTR_nRr_rpm]  "<MTR_nRr_rpm>"
  Bus Selector1/5 -> [MTR_TRrMtr_Nm]  "<MTR_TRrMtr_Nm>"
  Add6/1 -> Scope/2, Discrete-Time Integrator1/1
  Saturation2/1 -> Add5/2
  Saturation/1 -> Add5/1
  Add5/1 -> Scope/1, Discrete-Time Integrator/1
  Saturation1/1 -> Add6/1
  Saturation3/1 -> Add6/2
  [INV_PwrIn_W] -> Saturation/1
  [INV_PwrOut_W] -> Saturation2/1
  [INV_PwrOut_W] -> Saturation3/1
  [INV_PwrIn_W] -> Saturation1/1
  Discrete-Time Integrator/1 -> [INV_ELossesDsch_kWh]
  Discrete-Time Integrator1/1 -> [INV_ELossesChrg_kWh]
  Bus Selector3/1 -> [VCU_rSplitT]  "<VCU_rSplitT>"
  [INV_PMxDschFrt_W] -> INV_Fr/4
  [INV_PMxChrgFrt_W] -> INV_Fr/5
  Delay4/1 -> Gain/1
  [MTR_TFrtMtr_Nm] -> Delay4/1
  [MTR_PElecFrt_W] -> Gain7/1
  [MTR_nFrt_rpm] -> INV_Fr/3
  [INV_VEst_V] -> Bus Creator/6  "INV_VEst_V"
  [INV_rEffFrt] -> Bus Creator/7  "INV_rEffFrt"
  [INV_rEffRr] -> Bus Creator/8  "INV_rEffRr"
  [INV_PMxDschAct_W] -> Bus Creator/11  "INV_PMxDsch_W"
  [INV_PMxChrgAct_W] -> Bus Creator/12  "INV_PMxChrg_W"
  [INV_ELossesDsch_kWh] -> Bus Creator/13  "INV_ELossesDsch_kWh"
  [INV_ELossesChrg_kWh] -> Bus Creator/14  "INV_ELossesChrg_kWh"
  INV_Fr/1 -> [INV_rEffFrt]
  INV_Fr/4 -> [INV_PMxDschActFrt_W]
  INV_Fr/5 -> [INV_PMxChrgActFrt_W]
  INV_Fr/3 -> Gain4/1
  Gain/1 -> INV_Fr/1
  [INV_TMxFr_degC] -> Bus Creator/15  "INV_TMxFr_degC"
  [INV_TWtrOutFr_degC] -> Bus Creator/16  "INV_TWtrOutFr_degC"
  [INV_TMxRr_degC] -> Bus Creator/17  "INV_TMxRr_degC"
  [INV_TWtrOutRr_degC] -> Bus Creator/18  "INV_TWtrOutRr_degC"
  CS/1 -> Bus Selector2/1
  Bus Selector2/1 -> [INIT_TSys_degC]  "<INIT_TSys_degC>"
  Bus Selector2/2 -> [fEDU_PUMPdm]  "<fEDU_PUMPdm>"
  Bus Selector2/4 -> [CS_RAD_TWtrOut_degC]  "<CS_RAD_TWtrOut_degC>"
  [CS_RAD_TWtrOut_degC] -> INV_Fr/8
  [INIT_TSys_degC] -> INV_Fr/6
  Bus Selector2/3 -> [rEDU_PUMPdm]  "<rEDU_PUMPdm>"
  [MTR_TRrMtr_Nm] -> Delay1/1
  Delay1/1 -> Gain1/1
  Gain1/1 -> INV_Rr/1
  [INIT_TSys_degC] -> INV_Rr/6
  [rEDU_PUMPdm] -> Gain3/1
  [CS_RAD_TWtrOut_degC] -> INV_Rr/8
  [MTR_nRr_rpm] -> INV_Rr/3
  INV_Rr/3 -> Gain9/1
  INV_Rr/1 -> [INV_rEffRr]
  [INV_VEst_V] -> INV_Fr/9
  INV_Fr/6 -> [INV_TWtrOutFr_degC]
  [INV_VEst_V] -> INV_Rr/9
  INV_Rr/6 -> [INV_TWtrOutRr_degC]
  Gain2/1 -> INV_Fr/7
  Gain3/1 -> INV_Rr/7
  [fEDU_PUMPdm] -> Gain2/1
  [VCU_rSplitT] -> Divide2/1, Divide4/2
  [DC_PMxChrg_W] -> Divide1/2
  Divide1/1 -> [INV_PMxChrgFrt_W]
  [DC_PMxChrg_W] -> Divide2/2
  Divide2/1 -> [INV_PMxChrgRr_W]
  [VCU_rSplitT] -> Subtract2/1
  Constant2/1 -> Subtract2/2
  Subtract2/1 -> Divide3/2, Divide1/1
  Gain4/1 -> [INV_PLossFrt_W]
  INV_Fr/2 -> Gain8/1
  Max/1 -> [INV_TMxFr_degC]
  INV_Fr/7 -> Scope2/1, Max/1
  INV_Fr/8 -> Scope2/2, Max/2
  INV_Rr/7 -> Scope3/1, Max1/1
  INV_Rr/8 -> Scope3/2, Max1/2
  Max1/1 -> [INV_TMxRr_degC]
  Gain5/1 -> INV_Rr/2
  Gain6/1 -> [INV_PRr_W]
  Gain7/1 -> INV_Fr/2
  Gain8/1 -> [INV_PFr_W]
  Gain9/1 -> [INV_PLossRr_W]
  [INV_PLossFrt_W] -> Bus Creator/9  "INV_PLossFrt_W"
  [INV_PLossRr_W] -> Bus Creator/10  "INV_PLossRr_W"
  [INV_PFr_W] -> Add2/1
  [INV_PRr_W] -> Add2/2
  [INV_PLossFrt_W] -> Gain10/1
  Gain10/1 -> Terminator/1  "INV_Fr_HR_kW"
  [INV_PLossRr_W] -> Gain11/1
  Gain11/1 -> Terminator1/1  "INV_Rr_HR_kW"

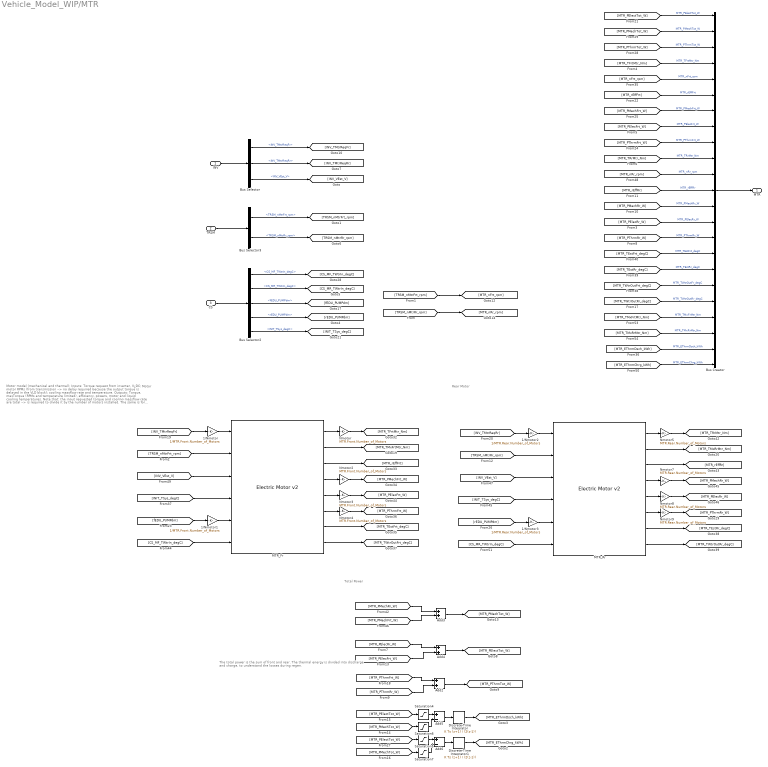
== system Vehicle_Model_WIP/MTR ==
  note: Rear Motor
  note: Front Motor
  note: Motor model (mechanical and thermal):
      | Inputs: Torque request from inverter, V_DC, motor RPMs (from transmission --> no delay required because the output torque is delayed in the VLD block); cooling massflow rate and temperature.
      | Outputs: Torque, maxTorque (RPMs and temperature limited), efficiency, powers, motor and liquid cooling temperatures.
      |
      | Note that: the input requested torque and cooling massflow rate are total --> is required to divide it by the number of motors installed. The same is for the output --> the total torque and the powers must be multiplied by the number of the motors.
      |
      | In case of lateral dynamics and Torque vectoring, the motor models number should match the real motor number.
  note: Total Power
  note: The total power is the sum of front and rear.
      |
      | The thermal energy is divided into discharge and charge, to understand the losses during regen.
  INV : Inport
  TRSM : Inport  Port=2
  CS : Inport  Port=3
  1/Nmotor : Gain  Gain=1/MTR.Front.Number_of_Motors
  1/Nmotor1 : Gain  Gain=1/MTR.Front.Number_of_Motors
  1/Nmotor2 : Gain  Gain=1/MTR.Rear.Number_of_Motors
  1/Nmotor3 : Gain  Gain=1/MTR.Rear.Number_of_Motors
  Add2 : Sum
  Add3 : Sum
  Add4 : Sum
  Add5 : Sum  Inputs=+-
  Add6 : Sum  Inputs=+-
  Bus Creator : BusCreator  Inputs=23
  Bus Selector : BusSelector  OutputSignals=INV_TMtrReqFr,INV_TMtrReqRr,INV_VEst_V
  Bus Selector2 : BusSelector  OutputSignals=CS_MF_TWtrIn_degC,CS_MR_TWtrIn_degC,fEDU_PUMPdm,rEDU_PUMPdm,INIT_TSys_degC
  Bus Selector3 : BusSelector  OutputSignals=TRSM_nMtrFrt_rpm,TRSM_nMtrRr_rpm
  Discrete-Time Integrator : DiscreteIntegrator  IntegratorMethod=Integration: Trapezoidal  gainval=1e-3/3600  SampleTime=-1  ICPrevOutput=DiscIntNeverNeededParam  ICPrevScaledInput=DiscIntNeverNeededParam
  Discrete-Time Integrator1 : DiscreteIntegrator  IntegratorMethod=Integration: Trapezoidal  gainval=1e-3/3600  SampleTime=-1  ICPrevOutput=DiscIntNeverNeededParam  ICPrevScaledInput=DiscIntNeverNeededParam
  MTR_Fr : EV_ePWT/Electric Motor v2  Mass_w=MTR.Front.Weigth_kg*0.5  cp_w=MTR.Front.cp_JpkgpK  Mass_s=MTR.Front.Weigth_kg  cp_s=MTR.Front.cp_JpkgpK  ThrmRtos=MTR.Front.ThrmR_KpW*0.42  MaxT=MTR.Front.TempMx_degC  RPM_bp1=MTR.Front.bp_RPM  voltage_bp=MTR.Front.bp_V  Torque_map=MTR.Front.Torque_Nm(:,:,1)  RPM_bp2=[1000 2000]  torque_bp=[100 200]  temp_bp=[25 35]  Efficiency_map=ones(2,2,2)*0.95  PL_torque_bp=MTR.Front.PLoss_T_bp  PL_RPM_bp=MTR.Front.PLoss_n_bp  PL_V_bp=MTR.Front.PLoss_V_bp  PL_map=MTR.Front.PLoss_table  D_h=13.33e-3  A_n=2e-4  lpm_tar=5  R_tar=MTR.Front.ThrmR_KpW*0.58  thermal_mode=from power losses maps
  MTR_Rr : EV_ePWT/Electric Motor v2  Mass_w=MTR.Rear.Weigth_kg*0.4  cp_w=MTR.Rear.cp_JpkgpK  Mass_s=MTR.Rear.Weigth_kg*0.5  cp_s=MTR.Rear.cp_JpkgpK  ThrmRtos=MTR.Rear.ThrmR_KpW*0.42  MaxT=MTR.Rear.TempMx_degC  RPM_bp1=MTR.Rear.bp_RPM  voltage_bp=MTR.Rear.bp_V  Torque_map=MTR.Rear.Torque_Nm(:,:,1)  RPM_bp2=[1000 2000]  torque_bp=[100 200]  temp_bp=[25 35]  Efficiency_map=ones(2,2,2)*0.95  PL_torque_bp=MTR.Rear.PLoss_T_bp  PL_RPM_bp=MTR.Rear.PLoss_n_bp  PL_V_bp=MTR.Rear.PLoss_V_bp  PL_map=MTR.Rear.PLoss_table  D_h=13.33e-3  A_n=2e-4  lpm_tar=10  R_tar=MTR.Rear.ThrmR_KpW*0.58  thermal_mode=from power losses maps
  Nmotor{,2..4} (4 alike) : Gain  Gain=MTR.Front.Number_of_Motors
  Nmotor{5,7..9} (4 alike) : Gain  Gain=MTR.Rear.Number_of_Motors
  Saturation4 : Saturate  UpperLimit=inf  LowerLimit=0
  Saturation5 : Saturate  UpperLimit=0  LowerLimit=-inf
  Saturation6 : Saturate  UpperLimit=inf  LowerLimit=0
  Saturation7 : Saturate  UpperLimit=0  LowerLimit=-inf
  MTR : Outport  VectorParamsAs1DForOutWhenUnconnected=off
  wires:
  INV/1 -> Bus Selector/1
  Bus Selector/3 -> [INV_VEst_V]  "<INV_VEst_V>"
  Bus Creator/1 -> MTR/1
  Bus Selector3/1 -> [TRSM_nMtrFrt_rpm]  "<TRSM_nMtrFrt_rpm>"
  Bus Selector3/2 -> [TRSM_nMtrRr_rpm]  "<TRSM_nMtrRr_rpm>"
  TRSM/1 -> Bus Selector3/1
  CS/1 -> Bus Selector2/1
  MTR_Rr/6 -> Nmotor9/1
  MTR_Fr/5 -> Nmotor3/1
  MTR_Rr/4 -> Nmotor7/1
  MTR_Fr/1 -> Nmotor/1
  MTR_Fr/6 -> Nmotor4/1
  MTR_Rr/1 -> Nmotor5/1
  MTR_Fr/4 -> Nmotor2/1
  [INV_VEst_V] -> MTR_Fr/3
  [INV_TMtrReqRr] -> 1/Nmotor2/1
  MTR_Rr/5 -> Nmotor8/1
  [TRSM_nMtrRr_rpm] -> MTR_Rr/2
  MTR_Fr/3 -> [MTR_rEffFrt]
  [INV_TMtrReqFr] -> 1/Nmotor/1
  [INV_VEst_V] -> MTR_Rr/3
  [TRSM_nMtrFrt_rpm] -> MTR_Fr/2
  Bus Selector/2 -> [INV_TMtrReqRr]  "<INV_TMtrReqRr>"
  Bus Selector/1 -> [INV_TMtrReqFr]  "<INV_TMtrReqFr>"
  MTR_Fr/8 -> [MTR_TWtrOutFrt_degC]
  [INIT_TSys_degC] -> MTR_Fr/4
  [fEDU_PUMPdm] -> 1/Nmotor1/1
  [CS_MF_TWtrIn_degC] -> MTR_Fr/6
  MTR_Fr/7 -> [MTR_TEstFrt_degC]
  [CS_MR_TWtrIn_degC] -> MTR_Rr/6
  MTR_Rr/8 -> [MTR_TWtrOutRr_degC]
  [rEDU_PUMPdm] -> 1/Nmotor3/1
  [INIT_TSys_degC] -> MTR_Rr/4
  MTR_Rr/7 -> [MTR_TEstRr_degC]
  [MTR_PMechFrt_W] -> Add3/2
  [MTR_PMechRr_W] -> Add3/1
  Add3/1 -> [MTR_PMechTot_W]
  [MTR_PElecRr_W] -> Add4/1
  [MTR_PElecFrt_W] -> Add4/2
  Add4/1 -> [MTR_PElectTot_W]
  [MTR_PThrmFrt_W] -> Add2/1
  [MTR_PThrmRr_W] -> Add2/2
  Add2/1 -> [MTR_PThrmTot_W]
  [MTR_PMechTot_W] -> Bus Creator/2  "MTR_PMechTot_W"
  [MTR_PElectTot_W] -> Bus Creator/1  "MTR_PElectTot_W"
  [MTR_PThrmTot_W] -> Bus Creator/3  "MTR_PThrmTot_W"
  [MTR_TFrtMtr_Nm] -> Bus Creator/4  "MTR_TFrtMtr_Nm"
  [MTR_rEffFrt] -> Bus Creator/6  "MTR_rEffFrt"
  [MTR_PMechFrt_W] -> Bus Creator/7  "MTR_PMechFrt_W"
  [MTR_PElecFrt_W] -> Bus Creator/8  "MTR_PElecFrt_W"
  [MTR_PThrmFrt_W] -> Bus Creator/9  "MTR_PThrmFrt_W"
  [MTR_TRrMtr_Nm] -> Bus Creator/10  "MTR_TRrMtr_Nm"
  [MTR_rEffRr] -> Bus Creator/12  "MTR_rEffRr"
  [MTR_PMechRr_W] -> Bus Creator/13  "MTR_PMechRr_W"
  [MTR_PElecRr_W] -> Bus Creator/14  "MTR_PElecRr_W"
  [MTR_PThrmRr_W] -> Bus Creator/15  "MTR_PThrmRr_W"
  [MTR_TEstFrt_degC] -> Bus Creator/16  "MTR_TEstFrt_degC"
  [MTR_TEstRr_degC] -> Bus Creator/17  "MTR_TEstRr_degC"
  [MTR_TWtrOutFrt_degC] -> Bus Creator/18  "MTR_TWtrOutFr_degC"
  [TRSM_nMtrFrt_rpm] -> [MTR_nFrt_rpm]
  [TRSM_nMtrRr_rpm] -> [MTR_nRr_rpm]
  [MTR_nFrt_rpm] -> Bus Creator/5  "MTR_nFrt_rpm"
  [MTR_nRr_rpm] -> Bus Creator/11  "MTR_nRr_rpm"
  [MTR_TMxFrtMtr_Nm] -> Bus Creator/20  "MTR_TMxFrMtr_Nm"
  [MTR_TMxRrMtr_Nm] -> Bus Creator/21  "MTR_TMxRrMtr_Nm"
  Add6/1 -> Discrete-Time Integrator1/1
  Saturation5/1 -> Add6/1
  Saturation4/1 -> Add5/1
  [MTR_PElectTot_W] -> Saturation4/1
  Add5/1 -> Discrete-Time Integrator/1
  [MTR_PMechTot_W] -> Saturation6/1
  Saturation6/1 -> Add5/2
  Saturation7/1 -> Add6/2
  [MTR_PElectTot_W] -> Saturation5/1
  [MTR_PMechTot_W] -> Saturation7/1
  [MTR_EThrmDsch_kWh] -> Bus Creator/22  "MTR_EThrmDsch_kWh"
  [MTR_EThrmChrg_kWh] -> Bus Creator/23  "MTR_EThrmChrg_kWh"
  Discrete-Time Integrator/1 -> [MTR_EThrmDsch_kWh]
  Discrete-Time Integrator1/1 -> [MTR_EThrmChrg_kWh]
  [MTR_TWtrOutRr_degC] -> Bus Creator/19  "MTR_TWtrOutRr_degC"
  Bus Selector2/1 -> [CS_MF_TWtrIn_degC]  "<CS_MF_TWtrIn_degC>"
  Bus Selector2/2 -> [CS_MR_TWtrIn_degC]  "<CS_MR_TWtrIn_degC>"
  Bus Selector2/3 -> [fEDU_PUMPdm]  "<fEDU_PUMPdm>"
  Bus Selector2/4 -> [rEDU_PUMPdm]  "<rEDU_PUMPdm>"
  1/Nmotor1/1 -> MTR_Fr/5
  1/Nmotor/1 -> MTR_Fr/1
  Nmotor/1 -> [MTR_TFrtMtr_Nm]
  MTR_Fr/2 -> [MTR_TMxFrtMtr_Nm]
  Nmotor2/1 -> [MTR_PMechFrt_W]
  Nmotor3/1 -> [MTR_PElecFrt_W]
  Nmotor4/1 -> [MTR_PThrmFrt_W]
  MTR_Rr/3 -> [MTR_rEffRr]
  1/Nmotor2/1 -> MTR_Rr/1
  1/Nmotor3/1 -> MTR_Rr/5
  Nmotor5/1 -> [MTR_TRrMtr_Nm]
  MTR_Rr/2 -> [MTR_TMxRrMtr_Nm]
  Nmotor7/1 -> [MTR_PMechRr_W]
  Nmotor8/1 -> [MTR_PElecRr_W]
  Nmotor9/1 -> [MTR_PThrmRr_W]
  Bus Selector2/5 -> [INIT_TSys_degC]  "<INIT_TSys_degC>"
